simulink model "sl_subsys_if1"  (Simulink 6.0)
settings: Solver=FixedStepDiscrete  StartTime=0.0  StopTime=10.0  FixedStep=1  RelTol=1e-3
settings Model: CovMetricSettings=d  Creator=The MathWorks Inc.  LastModifiedBy=batserve  ExtModeAutoUpdateStatusClock=off
settings OptimizationCC: BlockReduction=off  BooleanDataType=off
settings DebuggingCC: CheckExecutionContextPreStartOutputMsg=on  CheckExecutionContextRuntimeOutputMsg=on  SolverPrmCheckMsg=none
settings HardwareCC: TargetUnknown=on

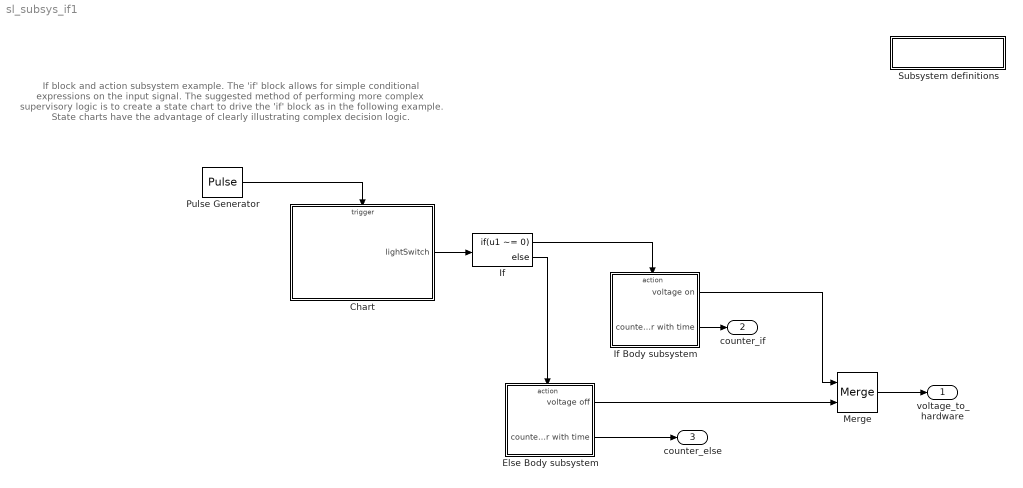
== system sl_subsys_if1 ==
  note: If block and action subsystem example.
      |
      | The 'if' block allows for simple conditional expressions on the input signal.
      | The suggested method of performing more complex supervisory logic is to
      | create a state chart to drive the 'if' block as in the following example.
      | State charts have the advantage of clearly illustrating complex decision
      | logic.
  " Subsystem definitions" : Subsystem  PropExecContextAcrossSSBoundary=on
      settings: OpenFcn=helpview([matlabroot,'/toolbox/simulink/simdemos/sl_subsys_definitions.html']);
      mask Display: disp('Subsystem\ndefinitions')
  Chart : Stateflow chart  TreatAsAtomicUnit=on  PropExecContextAcrossSSBoundary=on
  Else Body subsystem : Subsystem  TreatAsAtomicUnit=on  PropExecContextAcrossSSBoundary=on
  If : If  IfExpression=u1 ~= 0
  If Body subsystem : Subsystem  TreatAsAtomicUnit=on  PropExecContextAcrossSSBoundary=on
  Merge : Merge
  Pulse Generator : DiscretePulseGenerator
  voltage_to_hardware : Outport
  counter_if : Outport  Port=2
  counter_else : Outport  Port=3
  wires:
  Pulse Generator/1 -> Chart/Trigger
  Chart/1(lightSwitch) -> If/1
  If/1 -> If Body subsystem/Action
  If/2 -> Else Body subsystem/Action
  If Body subsystem/1(voltage on) -> Merge/1
  Else Body subsystem/1(voltage off) -> Merge/2
  Merge/1 -> voltage_to_hardware/1
  If Body subsystem/2(counter with time) -> counter_if/1
  Else Body subsystem/2(counter with time) -> counter_else/1

== system sl_subsys_if1/ Subsystem definitions ==

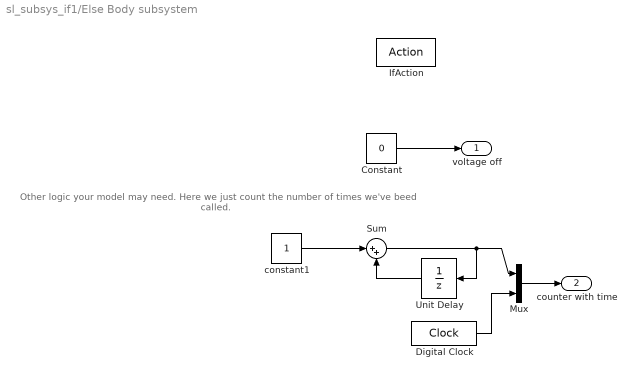
== system sl_subsys_if1/Else Body subsystem ==
  note: Other logic your model may need. Here we just count the number
      | of times we've beed called.
  IfAction : ActionPort  ActionType=else
  Constant : Constant  Value=0
  Digital Clock : DigitalClock
  Mux : Mux  Inputs=2
  Sum : Sum  Inputs=|++  SaturateOnIntegerOverflow=on  InputSameDT=on
  Unit Delay : UnitDelay  Orientation=left
  constant1 : Constant
  voltage off : Outport
  counter with time : Outport  Port=2
  wires:
  Constant/1 -> voltage off/1
  Sum/1 -> Mux/1, Unit Delay/1
  constant1/1 -> Sum/1
  Unit Delay/1 -> Sum/2
  Mux/1 -> counter with time/1
  Digital Clock/1 -> Mux/2

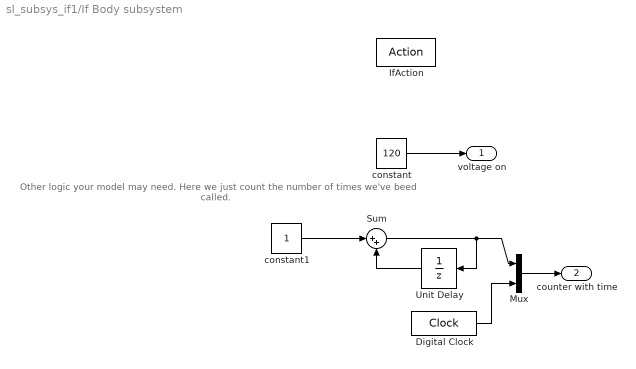
== system sl_subsys_if1/If Body subsystem ==
  note: Other logic your model may need. Here we just count the number
      | of times we've beed called.
  IfAction : ActionPort  ActionType=then
  Digital Clock : DigitalClock
  Mux : Mux  Inputs=2
  Sum : Sum  Inputs=|++  SaturateOnIntegerOverflow=on  InputSameDT=on
  Unit Delay : UnitDelay  Orientation=left
  constant : Constant  Value=120
  constant1 : Constant
  voltage on : Outport
  counter with time : Outport  Port=2
  wires:
  constant/1 -> voltage on/1
  Sum/1 -> Unit Delay/1, Mux/1
  constant1/1 -> Sum/1
  Unit Delay/1 -> Sum/2
  Mux/1 -> counter with time/1
  Digital Clock/1 -> Mux/2

== stateflow chart Chart ==
  state on
  state off
  on -> off : switch/lightSwitch=0;
  off -> on : switch/lightSwitch=1;
  (default) -> off : /lightSwitch=0;
  data: lightSwitch output double
  events: switch input EITHER_EDGE_EVENT
